simulink model "Sim02_TrackingDiff"  (R2020a)
settings: Solver=FixedStepAuto  StartTime=0.0  StopTime=T  FixedStep=Ts  RelTol=1e-3
values from neighbouring files (symbols this model uses):
  A = 1    [Sim02_Differentiator.m]    (also in Sim03_Differentiator.m)
  omg = 1    [Sim02_Differentiator.m]    (also in Sim03_Differentiator.m = 2*pi*f(k))
  Ts = 1e-3    (= 0.001)    [Sim01_Stability.m]    (also in Sim02_Differentiator.m = 1e-05; Sim03_Differentiator.m = 0.0001)
  umax = 1    [Sim01_Stability.m]    (also in Sim02_Differentiator.m = 20)
  xn = 0.1    [Sim02_Differentiator.m]    (also in Sim03_Differentiator.m)
  xnFlag = 1    [Sim02_Differentiator.m]    (also in Sim03_Differentiator.m = 0)
libraries: simulink x1
settings Model: Creator=XiaoCY  LastModifiedBy=XiaoCY
settings DataIOCC: ReturnWorkspaceOutputs=off

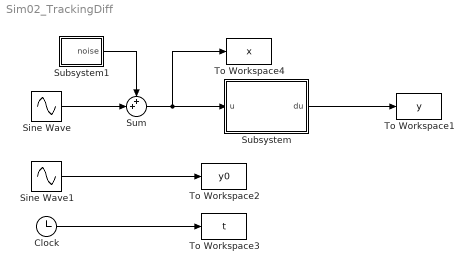
== system Sim02_TrackingDiff ==
  Clock : Clock
  Sine Wave : Sin  Amplitude=A  Frequency=omg  SampleTime=0
  Sine Wave1 : Sin  Amplitude=A  Frequency=omg  Phase=pi/2  SampleTime=0
  Subsystem : Subsystem
      mask Display: disp('Tracking\n\nDifferentiator')
  Subsystem1 : Subsystem
  Sum : Sum  Inputs=++|
  To Workspace1 : ToWorkspace  VariableName=y  SampleTime=Ts
  To Workspace2 : ToWorkspace  VariableName=y0  SampleTime=Ts
  To Workspace3 : ToWorkspace  VariableName=t  SampleTime=Ts
  To Workspace4 : ToWorkspace  VariableName=x  SampleTime=Ts
  wires:
  Clock/1 -> To Workspace3/1
  Sine Wave/1 -> Sum/2
  Sum/1 -> To Workspace4/1, Subsystem/1(u)
  Subsystem/1(du) -> To Workspace1/1
  Sine Wave1/1 -> To Workspace2/1
  Subsystem1/1(noise) -> Sum/1

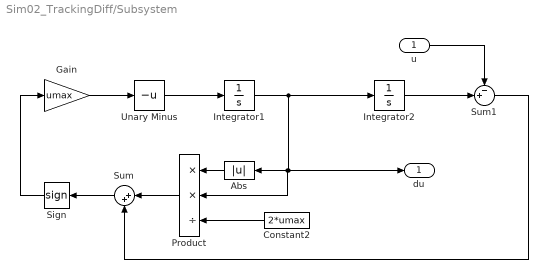
== system Sim02_TrackingDiff/Subsystem ==
  u : Inport
  Abs : Abs
  Constant2 : Constant  Value=2*umax
  Gain : Gain  Gain=umax
  Integrator1 : Integrator
  Integrator2 : Integrator
  Product : Product  Inputs=**/
  Sign : Signum
  Sum : Sum  Inputs=|++
  Sum1 : Sum  Inputs=-+|
  Unary Minus : UnaryMinus
  du : Outport
  wires:
  Abs/1 -> Product/1
  u/1 -> Sum1/1
  Integrator1/1 -> du/1, Product/2, Abs/1, Integrator2/1
  Sum/1 -> Sign/1
  Constant2/1 -> Product/3
  Product/1 -> Sum/1
  Unary Minus/1 -> Integrator1/1
  Sign/1 -> Gain/1
  Integrator2/1 -> Sum1/2
  Gain/1 -> Unary Minus/1
  Sum1/1 -> Sum/2

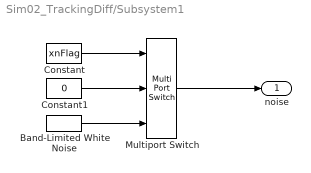
== system Sim02_TrackingDiff/Subsystem1 ==
  Band-Limited White Noise : simulink/Sources/Band-Limited White Noise  Cov=xn^2*Ts  Ts=Ts  seed=[23341]
  Constant : Constant  Value=xnFlag
  Constant1 : Constant  Value=0
  Multiport Switch : MultiPortSwitch  DataPortOrder=Zero-based contiguous  Inputs=2  zeroidx=on
  noise : Outport
  wires:
  Band-Limited White Noise/1 -> Multiport Switch/3
  Constant1/1 -> Multiport Switch/2
  Multiport Switch/1 -> noise/1
  Constant/1 -> Multiport Switch/1
